simulink model "ASG_collision_avoidance"  (R2024a)
settings: Solver=ode1  StartTime=0.0  StopTime=30  FixedStep=0.01  RelTol=1e-3
libraries: simulink x3
(part 1 of 3)
settings Model: Creator=victo  LastModifiedBy=victo

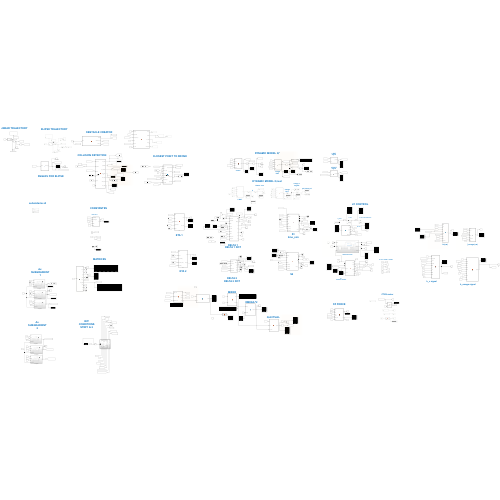
[thumbnail: Simulink's stored preview of the top-level diagram]
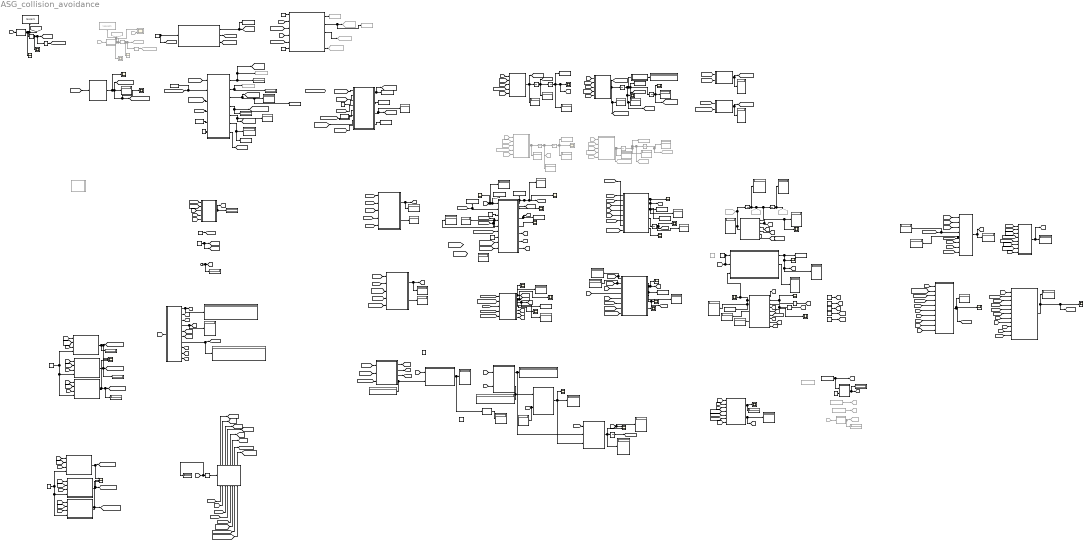
== system ASG_collision_avoidance ==
  note: LOW PASS FILTER
  note: DYNAMIC MODEL Q real
  note: h_omega signal
  note: ANGLES FOR ELIPSE
  note: CONSTANTES
  note: Av. SUBGRADIENT 2
  note: DELTA 1
      | DELTA 1 DOT
  note: ETA 2
  note: ELIPSE TRAJECTORY
  note: S2
  note: U1
      | CONTROL SIGNAL
  note: S1
  note: ETA 1
  note: h_v signal
  note: U1 CONTROL
  note: RHO & K1
  note: S1
      | time_sim
  note: q_dot
  note: f_omega(v,w)
  note: S1
  note: INIT CONDITIONS
      | STEP1 & 2
  note: MATRICES
  note: omega DOT
  note: V DOT
  note: V DOT
  note: Av. SUBGRADIENT 1
  note: omega DOT
  note: Q = Q*
  note: K1, K2, THETA1, THETA2
  note: DYNAMIC MODEL Q*
  note: Kappa - pos
  note: omega, v angular
  note: phi, theta, psi
  note: q = [x,y,z,phi,theta,psi]
  note: q_ddot
  note: subsistema s3
  note: MIXER
  note: OMEGA^2
  note: CTES motor
  note: fv(v,w)
  note: q DOT signal
  note: Q ACTUAL
  note: FZ FORCE
  note: q DDOT signal
  note: V
  note: OBSTACLE CREATOR
  note: COLLISION DETECTION
  note: DELTA 2
      | DELTA 2 DOT
  note: LINEAR TRAJECTORY
  note: CLOSEST POINT TO DRONE
  AverageBlock : Subsystem
  AverageBlock1 : Subsystem
  AverageBlock2 : Subsystem
  AverageBlock3 : Subsystem
  AverageBlock4 : Subsystem
  AverageBlock5 : Subsystem
  Clock : Clock
  Compare To Constant : simulink/Logic and Bit Operations/Compare To Constant  relop===  const=0.0  OutDataTypeStr=boolean
  Constant : Constant  Value=0.5
  Constant1 : Constant  Value=[0;0;0]
  Constant{9..10,19..20} (4 alike) : Constant
  Constant11 : Constant  Value=7
  Constant12 : Constant  Value=pi/4
  Constant13 : Constant  Value=1e-6
  Constant14 : Constant  Commented=on  Value=2*10^(-4)
  Constant15 : Constant  Commented=on  Value=1.95*10^(-4)  VectorParams1D=off
  Constant16 : Constant  Value=5  VectorParams1D=off
  Constant17 : Constant  Commented=on  Value=6*10^(-4)
  Constant18 : Constant  Value=5
  Constant2 : Constant  Value=[1;1;1;1]
  Constant21 : Constant  Value=90
  Constant22 : Constant  Value=7
  Constant3 : Constant  Value=[0;0;6;0;0;0]
  Constant4 : Constant  Value=5  VectorParams1D=off
  Constant5 : Constant  Value=0.03
  Constant6 : Constant  Value=45
  Constant7 : Constant  Value=6*10^(-3)
  Constant8 : Constant  Value=5
  DELTA 1 : Scope
  DELTA 2 : Scope
  DELTA1_DOT : Scope
  DELTA2 DOT4 : Scope
  Derivative1 : Derivative  Commented=on
  Derivative2 : Derivative  Commented=on
  Derivative3 : Derivative
  Derivative4 : Derivative
  Display{,1..54,56..62,64..65,67..69,71,89} (69 alike) : Display
  Display{55,70,73..75,77..78} (7 alike) : Display  Commented=on
  Enabled Subsystem : Subsystem  TreatAsAtomicUnit=on
  From100 : From  Commented=on  GotoTag=KAPPA
  From125 : From  Commented=on  GotoTag=FV
  From126 : From  Commented=on  GotoTag=ZERO_I
  From133 : From  Commented=on  GotoTag=TIME
  From134 : From  Commented=on  GotoTag=I_ZERO
  From146 : From  Commented=on  GotoTag=D_INV
  From147 : From  Commented=on  GotoTag=Q_ACTUAL
  From148 : From  Commented=on  GotoTag=XIsubk
  From157 : From  Commented=on  GotoTag=FW
  From199 : From  Commented=on  GotoTag=JM
  From217 : From  Commented=on  GotoTag=D_INV
  From218 : From  Commented=on  GotoTag=Q_ACTUAL
  From219 : From  Commented=on  GotoTag=XIsubk
  Fz : Scope
  Goto103 : Goto  Commented=on  GotoTag=DM
  Goto104 : Goto  Commented=on  GotoTag=JM
  Goto105 : Goto  Commented=on  GotoTag=JM_INV
  Goto138 : Goto  Commented=on  GotoTag=ANGLES_Q_DOT
  Goto139 : Goto  Commented=on  GotoTag=ANGLES_Q_DDOT
  Goto140 : Goto  Commented=on  GotoTag=V_LIN
  Goto37 : Goto  Commented=on  GotoTag=q_signal
  Goto38 : Goto  Commented=on  GotoTag=q_dot_signal
  Goto47 : Goto  Commented=on  GotoTag=ANGLES_Q
  Goto63 : Goto  Commented=on  GotoTag=q_ddot_signal
  Goto72 : Goto  Commented=on  GotoTag=V_DESEADA
  Goto73 : Goto  Commented=on  GotoTag=KAPPA_TRY
  Goto74 : Goto  Commented=on  GotoTag=V_DOT_DESEADA
  Goto84 : Goto  Commented=on  GotoTag=XI_VALUE
  Goto85 : Goto  Commented=on  GotoTag=OBS_unit_vector
  Goto89 : Goto  Commented=on  GotoTag=CENTER_closest
  HV : Scope
  HW : Scope
  Integrator{,1..6} (7 alike) : Integrator
  Integrator{9..12} (4 alike) : Integrator  Commented=on
  KAPPA : Scope
  KAPPA POS DESEADA : Scope  Commented=on
  KAPPA POS DESEADA1 : Scope
  KAPPA REAL1 : Scope
  KAPPA REAL2 : Scope  Commented=on
  KAPPA des : Scope  Commented=on  NumInputPorts=2
  MATLAB Function : MATLAB Function  TreatAsAtomicUnit=on
  MATLAB Function1 : MATLAB Function  TreatAsAtomicUnit=on
  MATLAB Function10 : MATLAB Function  TreatAsAtomicUnit=on
  MATLAB Function11 : MATLAB Function  TreatAsAtomicUnit=on
  MATLAB Function12 : MATLAB Function  TreatAsAtomicUnit=on
  MATLAB Function13 : MATLAB Function  TreatAsAtomicUnit=on
  MATLAB Function14 : MATLAB Function  TreatAsAtomicUnit=on
  MATLAB Function15 : MATLAB Function  TreatAsAtomicUnit=on
  MATLAB Function16 : MATLAB Function  TreatAsAtomicUnit=on
  MATLAB Function17 : MATLAB Function  TreatAsAtomicUnit=on
  MATLAB Function18 : MATLAB Function  TreatAsAtomicUnit=on
  MATLAB Function19 : MATLAB Function  TreatAsAtomicUnit=on
  MATLAB Function2 : MATLAB Function  TreatAsAtomicUnit=on
  MATLAB Function20 : MATLAB Function  Commented=on  TreatAsAtomicUnit=on
  MATLAB Function21 : MATLAB Function  TreatAsAtomicUnit=on
  MATLAB Function22 : MATLAB Function  TreatAsAtomicUnit=on
  MATLAB Function23 : MATLAB Function  TreatAsAtomicUnit=on
  MATLAB Function24 : MATLAB Function  TreatAsAtomicUnit=on
  MATLAB Function25 : MATLAB Function  TreatAsAtomicUnit=on
  MATLAB Function26 : MATLAB Function  Commented=on  TreatAsAtomicUnit=on
  MATLAB Function27 : MATLAB Function  TreatAsAtomicUnit=on
  MATLAB Function28 : MATLAB Function  Commented=on  TreatAsAtomicUnit=on
  MATLAB Function29 : MATLAB Function  TreatAsAtomicUnit=on
  MATLAB Function3 : MATLAB Function  TreatAsAtomicUnit=on
  MATLAB Function30 : MATLAB Function  TreatAsAtomicUnit=on
  MATLAB Function31 : MATLAB Function  TreatAsAtomicUnit=on
  MATLAB Function32 : MATLAB Function  TreatAsAtomicUnit=on
  MATLAB Function33 : MATLAB Function  TreatAsAtomicUnit=on
  MATLAB Function4 : MATLAB Function  TreatAsAtomicUnit=on
  MATLAB Function45 : MATLAB Function  TreatAsAtomicUnit=on
  MATLAB Function5 : MATLAB Function  Commented=on  TreatAsAtomicUnit=on
  MATLAB Function6 : MATLAB Function  TreatAsAtomicUnit=on
  MATLAB Function7 : MATLAB Function  TreatAsAtomicUnit=on
  MATLAB Function8 : MATLAB Function  TreatAsAtomicUnit=on
  MATLAB Function9 : MATLAB Function  TreatAsAtomicUnit=on
  MIU1 : Constant  Value=0.02
  MIU2 : Constant  Commented=on  Value=0.1
  NORM D1 : Scope
  NORM S1 : Scope
  NORM S2 : Scope
  Norm D2 : Scope
  Q FILTRADA = Q ESTRELLA : Scope
  "Q SIGNAL " : Scope
  Q_comparing : Scope  NumInputPorts=2
  ROTORS VEL : Scope
  S1 : Scope
  S2 : Scope
  SIGN : Signum
  SIGN S1 : Scope
  SIGN S2 : Scope
  Scope : Scope
  Scope1 : Scope  NumInputPorts=3
  Scope2 : Scope  NumInputPorts=3
  Scope3 : Scope
  Scope4 : Scope
  Sign1 : Signum
  Subsystem : Subsystem
  Subsystem1 : Subsystem  Commented=on
  THETA DESIRED : Scope
  THETA DOT DESIRED : Scope
  To Workspace : ToWorkspace  VariableName=dronepos  SampleTime=-1
  To Workspace1 : ToWorkspace  VariableName=simout1  SampleTime=-1
  To Workspace10 : ToWorkspace  VariableName=u1  SaveFormat=Timeseries  SampleTime=-1
  To Workspace11 : ToWorkspace  Commented=on  VariableName=kappad1  SampleTime=-1
  To Workspace12 : ToWorkspace  VariableName=obstaculos  SampleTime=-1
  To Workspace13 : ToWorkspace  VariableName=q_star  SampleTime=-1
  To Workspace14 : ToWorkspace  Commented=on  VariableName=droneor1  SampleTime=-1
  To Workspace15 : ToWorkspace  Commented=on  VariableName=dronepos1  SampleTime=-1
  To Workspace16 : ToWorkspace  Commented=on  VariableName=collision  SampleTime=-1
  To Workspace17 : ToWorkspace  Commented=on  VariableName=idx_obstac  SampleTime=-1
  To Workspace18 : ToWorkspace  Commented=on  VariableName=collision  SampleTime=-1
  To Workspace19 : ToWorkspace  VariableName=kappad1  SampleTime=-1
  To Workspace2 : ToWorkspace  VariableName=s1  SampleTime=-1
  To Workspace20 : ToWorkspace  Commented=on  VariableName=idx_obstac  SampleTime=-1
  To Workspace21 : ToWorkspace  VariableName=forward_vector  SampleTime=-1
  To Workspace22 : ToWorkspace  VariableName=closest_point  SampleTime=-1
  To Workspace23 : ToWorkspace  VariableName=closest_point1  SampleTime=-1
  To Workspace24 : ToWorkspace  VariableName=collision  SampleTime=-1
  To Workspace25 : ToWorkspace  VariableName=idx_obstac  SampleTime=-1
  To Workspace3 : ToWorkspace  VariableName=time_sim  SampleTime=-1
  To Workspace4 : ToWorkspace  VariableName=kappad  SampleTime=-1
  To Workspace5 : ToWorkspace  VariableName=a1  SampleTime=-1
  To Workspace6 : ToWorkspace  VariableName=realkappa  SampleTime=-1
  To Workspace7 : ToWorkspace  VariableName=droneor  SampleTime=-1
  To Workspace8 : ToWorkspace  VariableName=a2  SampleTime=-1
  To Workspace9 : ToWorkspace  VariableName=s2  SampleTime=-1
  Unit Delay : UnitDelay  SampleTime=-1  HasFrameUpgradeWarning=on
  VEL DESEADA : Scope  Commented=on
  VEL DESEADA1 : Scope
  ZETA1 : Scope
  ZETA2 : Scope
  eta1 : MATLAB Function  TreatAsAtomicUnit=on
  eta2 : MATLAB Function  TreatAsAtomicUnit=on
  theta1 : Constant  Value=0.01
  theta2 : Constant  Value=0.5
  theta5 : Constant  Value=1e-6
  wires:
  [C_q] -> MATLAB Function/4(C_q)
  Integrator10/1 -> To Workspace14/1, Goto138/1, Integrator12/1, Display74/1
  [DESIRED_DTHETA_ELIP] -> MATLAB Function8/5(omega_desired)
  MATLAB Function15/1(R) -> [R3]
  MATLAB Function22/1(Q4x1) -> Display47/1
  [q_dot_signal] -> MATLAB Function24/4(q_dot)
  [A2X_AVERAGE] -> MATLAB Function19/6(a2x_average)
  Derivative2/1 -> Goto74/1
  From126/1 -> MATLAB Function28/2(zero_I)
  Enabled Subsystem/5(theta0) -> [THETA0]
  MATLAB Function24/2(Q4) -> [Q4], Display46/1
  [D_INV] -> MATLAB Function14/3(D_inv)
  [THETADOT_DES0] -> eta2/5(THETA_DOT_0)
  MATLAB Function18/1(h_omega) -> [H_OMEGA], HW/1, Display35/1
  [TIME] -> Compare To Constant/1, Display51/1
  MATLAB Function9/7(drag_matrix) -> Display53/1, [DRAG_MATRIX]
  MATLAB Function3/3(a1) -> [A1], To Workspace5/1
  [A1_Z] -> AverageBlock2/1(a1_z)
  MATLAB Function6/1(s1) -> Display10/1, To Workspace2/1, [S1], S1/1
  [D_INV] -> MATLAB Function10/2(D_inv)
  [Q4] -> Display49/1, MATLAB Function2/2(control4x1)
  [THETADOT0] -> eta2/4(THETA_DOT_desired_0)
  MATLAB Function9/9(M) -> [Masa]
  Subsystem/1(Q_STAR) -> [Q], Display64/1, Q FILTRADA = Q ESTRELLA/1, To Workspace13/1
  MATLAB Function3/1(delta1) -> DELTA 1/1, Display11/1, [DELTA1], To Workspace1/1
  [Q] -> MATLAB Function13/1(Q)
  Unit Delay/1 -> [Q_actual]
  From125/1 -> MATLAB Function5/1(fv)
  [V_ACTUAL] -> MATLAB Function45/1(v_lin)
  MATLAB Function13/1(Q_6X1) -> MATLAB Function22/1(Q6x1), Display32/1
  [KA] -> MATLAB Function9/1("Ka ")
  [D_INV] -> MATLAB Function/3(D_inv)
  From199/1 -> MATLAB Function26/1(Jm)
  [OMEGA_ACTV1] -> MATLAB Function45/2(v_ang)
  [DESIRED_DTHETA_ELIP] -> Enabled Subsystem/8(thetadot_desired)
  [THETA1] -> MATLAB Function16/5(theta1)
  Integrator4/1 -> MATLAB Function7/1(vector_rpy), Integrator6/1, To Workspace7/1, [OMEGA_ACTV1], Scope3/1, [ANGLES_Q_DOT], Display21/1
  MATLAB Function15/3(R_ddot) -> [R3_DDOT]
  [V_DESIRED0] -> eta1/3(v_deseada_0)
  MATLAB Function23/1(Q_actual) -> Unit Delay/1, Q_comparing/2, Display37/1
  [D_INV] -> MATLAB Function17/3(D_inv)
  [V_DOT_DESEADA] -> MATLAB Function16/2(v_dot_deseada)
  Enabled Subsystem/2(kappa0) -> [KAPPA_0]
  [V_ACTUAL] -> Enabled Subsystem/1(v_actual)
  Clock/1 -> Display52/1, [TIME]
  Enabled Subsystem/4(kappaD0) -> [KAPPAD0]
  MATLAB Function4/1(k1) -> Display12/1, [K1]
  [THETA2] -> MATLAB Function19/5(theta2)
  [ETA2] -> MATLAB Function18/4(eta2)
  [THETA2] -> AverageBlock5/2(theta)
  [FV] -> MATLAB Function14/1(fv)
  From133/1 -> MATLAB Function20/1(t)
  MATLAB Function28/1(omega_dot) -> Integrator10/1, Display75/1, Goto139/1
  [V_DESEADA] -> Enabled Subsystem/3(v_desired)
  [OMEGA_ACTV1] -> MATLAB Function11/5(omega)
  MATLAB Function12/3(value_s2) -> Display71/1
  MATLAB Function19/3(norm_s2) -> NORM S2/1
  [DRAG_MATRIX] -> MATLAB Function10/8(drag_matrix)
  MATLAB Function8/6(a2_y) -> [A2_Y]
  [V_ACTUAL] -> Display14/1, MATLAB Function3/4(v_actual)
  From148/1 -> MATLAB Function5/5(xi_subv)
  MATLAB Function19/2(Z2) -> [ZETA2], ZETA2/1
  MATLAB Function12/2(value_s1) -> Display68/1
  Constant10/1 -> AverageBlock3/4(constant sign), AverageBlock5/4(constant sign), AverageBlock4/4(constant sign)
  MATLAB Function8/5(a2_x) -> [A2_X]
  Integrator9/1 -> Goto140/1, Integrator11/1, Display70/1
  From157/1 -> MATLAB Function28/1(fw)
  [H_V] -> MATLAB Function12/5(h_v)
  MATLAB Function8/7(a2_z) -> [A2_Z]
  [Q] -> MATLAB Function18/10(Q)
  [TIME] -> AverageBlock1/3(t)
  MATLAB Function9/10(g) -> [G_cte]
  [DRAG_MATRIX] -> MATLAB Function/6(drag_matrix)
  Enabled Subsystem/7(theta_desired0) -> [THETA_DES0]
  [DELTA1] -> MATLAB Function6/1(delta1)
  MATLAB Function8/4(F_d2) -> Norm D2/1
  [ZERO_I] -> MATLAB Function17/2(zero_I)
  MATLAB Function8/2(delta2_dot) -> Display39/1, DELTA2 DOT4/1, [DELTA2_DOT]
  [G_Q] -> MATLAB Function11/6(g_q)
  Derivative1/1 -> VEL DESEADA/1, Goto72/1, Derivative2/1
  [KA] -> MATLAB Function24/3(Ka)
  From219/1 -> MATLAB Function28/5(xi_subw)
  [D] -> MATLAB Function12/1(D)
  [G_Q] -> MATLAB Function/5(g_q)
  [G_cte] -> MATLAB Function24/2(g)
  From147/1 -> MATLAB Function5/4(Q)
  MATLAB Function12/1(u1) -> To Workspace10/1, Display43/1, "Q SIGNAL "/1, Subsystem/3(U1)
  SIGN/1 -> MATLAB Function12/2(sign_s1), SIGN S1/1
  [A2_X] -> AverageBlock3/1(a2_x)
  [A2Z_AVERAGE] -> MATLAB Function19/8(a2z_average)
  [XIsubk] -> MATLAB Function4/1(xi_subkappa)
  [D_INV] -> MATLAB Function18/9(D_inv)
  [TIME] -> AverageBlock3/3(t)
  [Masa] -> MATLAB Function24/1(M)
  [TIME] -> MATLAB Function4/3(t)
  Integrator1/1 -> Display3/1, Goto37/1
  MATLAB Function20/1(kappa) -> KAPPA des/1, Derivative1/1, To Workspace11/1, Goto73/1, KAPPA POS DESEADA/1
  [A2_Y] -> AverageBlock4/1(In1)
  MATLAB Function9/8(l_arm) -> [L_ARM]
  [Q] -> Q_comparing/1, Display48/1
  [Q] -> MATLAB Function/2(Q), Scope/1, Display67/1
  [OMEGA_ACTV1] -> Display18/1, MATLAB Function10/5(omega)
  [V_ACT_0] -> eta1/2(v_0)
  [ZERO_I] -> MATLAB Function18/11(zero_I)
  [DELTA2] -> MATLAB Function18/3(delta2)
  [THETA1] -> AverageBlock1/2(theta)
  From100/1 -> KAPPA des/2
  [RHO1] -> MATLAB Function4/5(rho1)
  [V_ACTUAL] -> MATLAB Function11/4(v)
  [DELTA2] -> MATLAB Function19/1(delta2), Display7/1
  [V_DOT_ACTUAL] -> MATLAB Function25/1(v_lin)
  [V_ACTUAL] -> MATLAB Function16/3(v_actual)
  MATLAB Function25/1(q_dot_signal) -> Display44/1, [q_ddot_signal]
  [KAPPA_TRY] -> To Workspace4/1, MATLAB Function3/2(kappa_desired)
  [I_ZERO] -> MATLAB Function10/1(I_zero)
  AverageBlock5/1(Out1) -> [A2Z_AVERAGE], Scope2/3
  [ZETA2] -> MATLAB Function18/5(zeta2)
  MATLAB Function7/1(R_graph) -> Display26/1
  [THETA1] -> AverageBlock/2(theta)
  [TIME] -> MATLAB Function19/4(t)
  [A2] -> MATLAB Function18/8(a2)
  theta1/1 -> [THETA1]
  [EPSILON] -> MATLAB Function8/3(epsilon)
  eta1/1(eta1) -> [ETA1], Display5/1
  AverageBlock1/1(Out1) -> Scope1/2, Display29/1, [A1Y_AVERAGE]
  From146/1 -> MATLAB Function5/3(D_inv)
  MATLAB Function9/2(D_inv) -> [D_INV]
  [ANGLES_Q_DDOT] -> MATLAB Function25/2(v_ang)
  From134/1 -> MATLAB Function5/2(I_zero)
  [XIsubk] -> MATLAB Function17/5(xi_subw)
  Constant9/1 -> AverageBlock2/4(constant sign), AverageBlock1/4(constant sign), AverageBlock/4(constant sign)
  [G_Q] -> MATLAB Function10/6(g_q)
  [THETA1] -> MATLAB Function4/4(theta1)
  [KAPPA] -> Enabled Subsystem/2(kappa)
  [A1_X] -> AverageBlock/1(a1_x)
  [THETA_DES0] -> eta2/3(THETA_deseada_0)
  [DELTA2_DOT] -> Display65/1, MATLAB Function19/2(delta2_dot)
  AverageBlock4/1(Out1) -> [A2Y_AVERAGE], Scope2/2
  MATLAB Function9/5(I_zero) -> [I_ZERO]
  MATLAB Function1/2(mixer_inv) -> MATLAB Function2/1(mixer_inv), Display15/1
  [FW] -> MATLAB Function18/1(fw)
  [THETA1] -> AverageBlock2/2(theta)
  [DESIRED_THETA_ELIP] -> Enabled Subsystem/7(theta_desired)
  MATLAB Function10/1(fv) -> [FV], Display23/1
  eta2/2(sum_result) -> Display41/1
  [A2_Z] -> AverageBlock5/1(In1)
  [H_OMEGA] -> MATLAB Function12/6(h_omega)
  [KAPPA_0] -> eta1/5(kappa_0)
  MATLAB Function2/1(rotors_vel) -> MATLAB Function23/3(rotors_vel4x1), ROTORS VEL/1, Display34/1
  Constant1/1 -> [XIsubk], [XIsubk_dot]
  MATLAB Function9/4(g_q) -> Display27/1, [G_Q]
  MATLAB Function9/3(C) -> [C_q]
  [TIME] -> AverageBlock4/3(t)
  [Q] -> MATLAB Function17/4(Q)
  [DELTA1_DOT] -> MATLAB Function6/2(delta1_dot)
  [THETA0] -> eta2/2(THETA_0)
  From218/1 -> MATLAB Function28/4(Q)
  [Q] -> MATLAB Function14/4(Q)
  [FV] -> MATLAB Function16/1(fv)
  MATLAB Function6/4(norm_s1) -> NORM S1/1
  Integrator2/1 -> Display/1, ZETA1/1, [ZETA1]
  [XIsubk] -> MATLAB Function14/5(xi_subv)
  [FW] -> MATLAB Function17/1(fw)
  Integrator12/1 -> Goto47/1, Display77/1
  Subsystem/2(Q_DOT_STAR) -> Display69/1
  [q_ddot_signal] -> MATLAB Function24/5(q_ddot)
  [TIME] -> MATLAB Function18/7(t)
  [THETA_ACTUAL] -> MATLAB Function8/1(theta_actual)
  [THETA2] -> AverageBlock4/2(theta)
  AverageBlock2/1(Out1) -> Display1/1, [A1Z_AVERAGE], Scope1/3
  MATLAB Function21/1(desired_theta) -> THETA DESIRED/1, [DESIRED_THETA_ELIP], THETA DOT DESIRED/1, [DESIRED_DTHETA_ELIP], Display13/1
  MATLAB Function8/1(delta2) -> DELTA 2/1, Display38/1, [DELTA2]
  [S1] -> MATLAB Function12/8(s1)
  [TIME] -> AverageBlock2/3(t)
  [TIME] -> MATLAB Function16/10(t)
  MATLAB Function24/1(Fz) -> Display45/1, Fz/1
  [A1_Y] -> AverageBlock1/1(In1)
  MATLAB Function8/3(a2) -> To Workspace8/1, [A2]
  From217/1 -> MATLAB Function28/3(D_inv)
  MATLAB Function16/1(hv) -> [H_V], Display36/1, HV/1
  AverageBlock/1(Out1) -> Display33/1, [A1X_AVERAGE], Scope1/1
  [S1] -> SIGN/1
  Enabled Subsystem/8(thetadot_desired0) -> [THETADOT_DES0]
  [ETA1] -> MATLAB Function6/3(eta1)
  Enabled Subsystem/3(vdesired0) -> [V_DESIRED0]
  Enabled Subsystem/6(thetadot0) -> [THETADOT0]
  [KFC0] -> MATLAB Function11/8(Kf_c0)
  [DESIRED_THETA_ELIP] -> MATLAB Function8/2(theta_desired)
  [C_q] -> MATLAB Function11/3(C)
  [I_ZERO] -> MATLAB Function14/2(I_zero)
  [ANGLES_Q_DDOT] -> MATLAB Function15/3(anglesddot_vector)
  [XIsubk_dot] -> MATLAB Function4/2(xi_subkappa_dot)
  [OMEGA_ACTV1] -> MATLAB Function8/4(omega_actual)
  MATLAB Function5/1(v_dot) -> Integrator9/1, Display73/1
  [RHO2] -> MATLAB Function12/7(k2)
  MATLAB Function3/5(a1_x) -> [A1_X]
  [V_DESEADA] -> MATLAB Function3/5(v_desired), Display30/1
  [S2] -> Sign1/1
  [THETA2] -> eta2/1(theta2)
  [DELTA1] -> MATLAB Function16/8(delta1)
  eta2/1(eta2) -> [ETA2], Display40/1
  [A1X_AVERAGE] -> MATLAB Function6/6(a1x_average)
  MATLAB Function9/6(zero_I) -> [ZERO_I]
  [KAPPA_TRY] -> Enabled Subsystem/4(kappa_try)
  [ZETA1] -> MATLAB Function16/9(zeta1)
  [THETA1] -> eta1/1(theta1)
  MATLAB Function27/1(Km) -> Display50/1, [KM]
  [THETA_ACTUAL] -> Enabled Subsystem/5(theta_actual)
  MATLAB Function11/1(fw) -> Display19/1, [FW]
  MATLAB Function3/4(F_d1) -> NORM D1/1
  [THETA2] -> MATLAB Function18/6(theta2)
  [THETA2] -> AverageBlock3/2(theta)
  MATLAB Function3/6(a1_y) -> [A1_Y]
  MATLAB Function1/1(mixer) -> MATLAB Function23/2(mixer), Display8/1
  MATLAB Function15/4(R_inv) -> MATLAB Function13/2(R_inv), Display22/1
  MIU1/1 -> [MIU], Subsystem/2(MIU2), Subsystem/1(MIU1)
  Integrator/1 -> Display4/1, Goto38/1, MATLAB Function/1(q_dot), Integrator1/1
  [THETA_ACTUAL] -> MATLAB Function15/1(angles_vector)
  [ETA1] -> MATLAB Function16/7(eta1)
  Sign1/1 -> SIGN S2/1, MATLAB Function12/3(sign_s2)
  [DRAG_MATRIX] -> MATLAB Function11/7(drag_matrix)
  Integrator6/1 -> Scope4/1, [THETA_ACTUAL], Display28/1
  MATLAB Function17/1(omega_dot) -> [THETA_ACTUAL_DDOT], [ANGLES_Q_DDOT], Display25/1, Integrator4/1
  MATLAB Function14/1(v_dot) -> [V_DOT_ACTUAL], Display20/1, Integrator3/1
  [ANGLES_Q_DOT] -> MATLAB Function15/2(anglesdot_vector)
  [TIME] -> AverageBlock/3(t)
  MATLAB Function6/3(Z1) -> Integrator2/1
  eta1/2(sum_result) -> Display9/1
  [V_DESEADA] -> MATLAB Function21/1(des_vel)
  [OMEGA_ACTV1] -> Enabled Subsystem/6(omega_actual)
  Enabled Subsystem/1(v_actual0) -> [V_ACT_0]
  [TIME] -> AverageBlock5/3(t)
  [A2Y_AVERAGE] -> MATLAB Function19/7(a2y_average)
  AverageBlock3/1(Out1) -> [A2X_AVERAGE], Scope2/1
  MATLAB Function15/2(R_dot) -> [R3_DOT]
  theta2/1 -> [THETA2]
  [KV] -> MATLAB Function1/1(Kv)
  MATLAB Function45/1(q_dot_signal) -> Display89/1, [q_dot_signal]
  [KFC0] -> MATLAB Function10/7(kf_c0)
  Integrator11/1 -> To Workspace15/1, KAPPA REAL2/1, Display78/1
  [ZERO_I] -> MATLAB Function11/1(zero_I)
  [TIME] -> MATLAB Function6/4(t)
  [D_INV] -> MATLAB Function11/2(D_inv)
  [KM] -> MATLAB Function1/2(Km)
  Compare To Constant/1 -> Enabled Subsystem/Enable
  [A1Y_AVERAGE] -> MATLAB Function6/7(a1y_average)
  [KAPPA] -> KAPPA/1, Display6/1, To Workspace6/1, MATLAB Function3/1(kappa_actual)
  Integrator5/1 -> [KAPPA], KAPPA REAL1/1, Display31/1, To Workspace/1
  [OMEGA_ACTV1] -> MATLAB Function18/2(omega)
  MATLAB Function6/2(t_s1) -> To Workspace3/1
  [V_DESEADA] -> MATLAB Function16/4(v_deseada)
  Constant15/1 -> Goto104/1
  Constant7/1 -> MATLAB Function27/1(Kv), [KV]
  [A1Z_AVERAGE] -> MATLAB Function6/8(a1z_average)
  [C_q] -> MATLAB Function10/3(C)
  Integrator3/1 -> Integrator5/1, Display16/1, [V_ACTUAL]
  [Q] -> MATLAB Function24/7(Q6)
  MATLAB Function3/7(a1_z) -> [A1_Z]
  [K1] -> MATLAB Function12/4(k1)
  [V_ACTUAL] -> Display17/1, MATLAB Function10/4(v)
  MATLAB Function3/2(delta1_dot) -> [DELTA1_DOT], DELTA1_DOT/1
  MATLAB Function/1(out) -> Display2/1, Integrator/1, Goto63/1
  Constant14/1 -> Goto103/1
  MATLAB Function9/1(D) -> Display24/1, [D]
  [A1] -> MATLAB Function16/6(a1)
  MATLAB Function19/1(s2) -> Display42/1, To Workspace9/1, S2/1, [S2]
  theta5/1 -> [EPSILON]
  Constant4/1 -> [RHO2]
  MATLAB Function26/1(Jm_inv) -> Goto105/1, Display55/1
  [THETA1] -> MATLAB Function6/5(theta1)
  [S2] -> MATLAB Function12/9(s2)
  Constant5/1 -> MATLAB Function27/2(porcent_force)
  [ETA2] -> MATLAB Function19/3(eta2)
  [R3] -> MATLAB Function23/1(R)
  Constant/1 -> [KA]
  [KAPPAD0] -> eta1/4(kappa_desired_0)
  [THETA_ACTUAL] -> MATLAB Function24/6(theta_actual)
  MATLAB Function29/1(obstaculos) -> To Workspace12/1, [OBSTACLES]
  [KAPPA] -> MATLAB Function30/1(drone_center)
  [OBSTACLES] -> MATLAB Function30/3(obstacles)
  MATLAB Function30/1(hay_colision) -> [XI_VALUE], To Workspace16/1, Display54/1
  MATLAB Function30/2(idx_obstaculo) -> To Workspace17/1, Display56/1
  [XI_VALUE] -> MATLAB Function3/6(collision)
  Constant8/1 -> MATLAB Function3/7(gamma)
  MATLAB Function30/3(centro_obstaculo) -> To Workspace22/1, Display57/1, [CENTER_closest]
  Constant11/1 -> [MIN_DISTANCE], MATLAB Function30/2(max_distancia)
  MATLAB Function30/4(angulo_relativo) -> Display58/1, [OBST_angle]
  [TIME] -> MATLAB Function31/1(t)
  Derivative4/1 -> [V_DOT_DESEADA]
  Derivative3/1 -> VEL DESEADA1/1, [V_DESEADA], Derivative4/1
  MATLAB Function31/1(kappa) -> KAPPA POS DESEADA1/1, Derivative3/1, To Workspace19/1, [KAPPA_TRY]
  Constant12/1 -> MATLAB Function30/5(fov_angle)
  [THETA_ACTUAL] -> MATLAB Function30/4(drone_angles)
  MATLAB Function30/5(vector_centro) -> [OBS_unit_vector], Display59/1
  Constant13/1 -> MATLAB Function3/3(epsilon)
  Constant19/1 -> MATLAB Function30/6(Kd)
  Constant16/1 -> [RHO1]
  [V_ACTUAL] -> MATLAB Function32/2(kappa_derivative)
  Constant6/1 -> MATLAB Function32/1(FOV_angle)
  [KAPPA] -> MATLAB Function32/4(kappa)
  MATLAB Function29/3(radios_value) -> [RADIOS_VALUE]
  MATLAB Function29/2(obstacles_center_list) -> [OBS_CENTER_LIST]
  [OBS_CENTER_LIST] -> MATLAB Function32/3(obstaculos_center_list)
  [RADIOS_VALUE] -> MATLAB Function32/5(radio_value)
  Constant20/1 -> MATLAB Function32/6(drone_radio)
  MATLAB Function32/2(collision) -> To Workspace18/1, Goto84/1
  MATLAB Function32/1(idx_min) -> To Workspace20/1
  MATLAB Function32/3(unit_vector) -> Goto85/1
  MATLAB Function32/5(closest_center) -> Goto89/1
  MATLAB Function30/6(forward_vector) -> To Workspace21/1, Display60/1
  Constant18/1 -> MATLAB Function29/1(shifft1), [SHIFFT1]
  [KAPPA] -> MATLAB Function33/1(dron_pos)
  [SHIFFT1] -> MATLAB Function33/2(shifft1)
  MATLAB Function33/1(punto_mas_cercano) -> [CENTER_clst], To Workspace23/1
  MATLAB Function33/3(unitary_vector) -> Display62/1, [UNITARY_VEC]
  MATLAB Function33/4(hay_colision) -> To Workspace24/1
  MATLAB Function33/2(idx_obstaculo) -> To Workspace25/1
  [THETA_ACTUAL] -> MATLAB Function33/4(drone_angles)
  Constant21/1 -> MATLAB Function33/5(fov_angle)
  Constant22/1 -> MATLAB Function33/3(distancia_minima)
  [UNITARY_VEC] -> MATLAB Function3/9(unitary_vector)
  [CENTER_clst] -> MATLAB Function3/8(center_closest)
  [OBSTACLES] -> MATLAB Function33/6(obstaculos)
  [CENTER_closest] -> MATLAB Function33/7(center_closest_red)
  MATLAB Function30/7(aux_variable) -> [AUX_VAR]
  [AUX_VAR] -> MATLAB Function33/8(aux_variable)

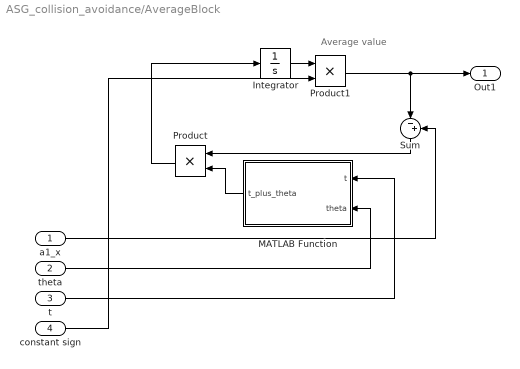
== system ASG_collision_avoidance/AverageBlock ==
  note: Average value
  a1_x : Inport
  theta : Inport  Port=2
  t : Inport  Port=3
  constant sign : Inport  Port=4
  Integrator : Integrator
  MATLAB Function : MATLAB Function  TreatAsAtomicUnit=on
  Product : Product
  Product1 : Product
  Sum : Sum  Inputs=|-+
  Out1 : Outport
  wires:
  MATLAB Function/1(t_plus_theta) -> Product/2
  Sum/1 -> Product/1
  Product/1 -> Integrator/1
  theta/1 -> MATLAB Function/2(theta)
  a1_x/1 -> Sum/2
  t/1 -> MATLAB Function/1(t)
  Integrator/1 -> Product1/1
  Product1/1 -> Out1/1, Sum/1
  constant sign/1 -> Product1/2

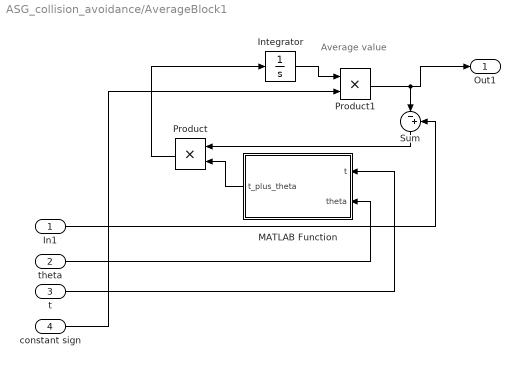
== system ASG_collision_avoidance/AverageBlock1 ==
  note: Average value
  In1 : Inport
  theta : Inport  Port=2
  t : Inport  Port=3
  constant sign : Inport  Port=4
  Integrator : Integrator
  MATLAB Function : MATLAB Function  TreatAsAtomicUnit=on
  Product : Product
  Product1 : Product
  Sum : Sum  Inputs=|-+
  Out1 : Outport
  wires:
  MATLAB Function/1(t_plus_theta) -> Product/2
  Sum/1 -> Product/1
  Product/1 -> Integrator/1
  theta/1 -> MATLAB Function/2(theta)
  In1/1 -> Sum/2
  t/1 -> MATLAB Function/1(t)
  Product1/1 -> Sum/1, Out1/1
  Integrator/1 -> Product1/1
  constant sign/1 -> Product1/2

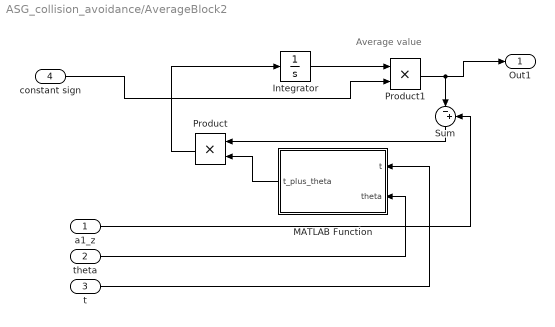
== system ASG_collision_avoidance/AverageBlock2 ==
  note: Average value
  a1_z : Inport
  theta : Inport  Port=2
  t : Inport  Port=3
  constant sign : Inport  Port=4
  Integrator : Integrator
  MATLAB Function : MATLAB Function  TreatAsAtomicUnit=on
  Product : Product
  Product1 : Product
  Sum : Sum  Inputs=|-+
  Out1 : Outport
  wires:
  MATLAB Function/1(t_plus_theta) -> Product/2
  Sum/1 -> Product/1
  Product/1 -> Integrator/1
  theta/1 -> MATLAB Function/2(theta)
  a1_z/1 -> Sum/2
  t/1 -> MATLAB Function/1(t)
  Integrator/1 -> Product1/1
  Product1/1 -> Sum/1, Out1/1
  constant sign/1 -> Product1/2

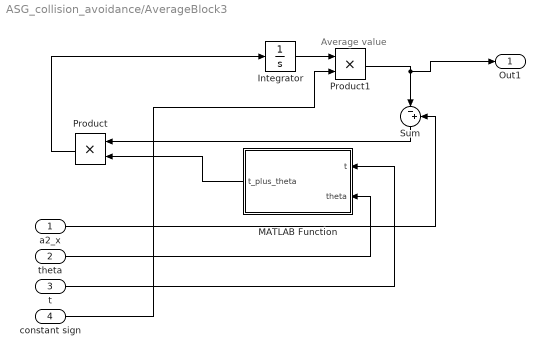
== system ASG_collision_avoidance/AverageBlock3 ==
  note: Average value
  a2_x : Inport
  theta : Inport  Port=2
  t : Inport  Port=3
  constant sign : Inport  Port=4
  Integrator : Integrator
  MATLAB Function : MATLAB Function  TreatAsAtomicUnit=on
  Product : Product
  Product1 : Product
  Sum : Sum  Inputs=|-+
  Out1 : Outport
  wires:
  MATLAB Function/1(t_plus_theta) -> Product/2
  Sum/1 -> Product/1
  Product/1 -> Integrator/1
  theta/1 -> MATLAB Function/2(theta)
  a2_x/1 -> Sum/2
  t/1 -> MATLAB Function/1(t)
  Integrator/1 -> Product1/1
  constant sign/1 -> Product1/2
  Product1/1 -> Sum/1, Out1/1

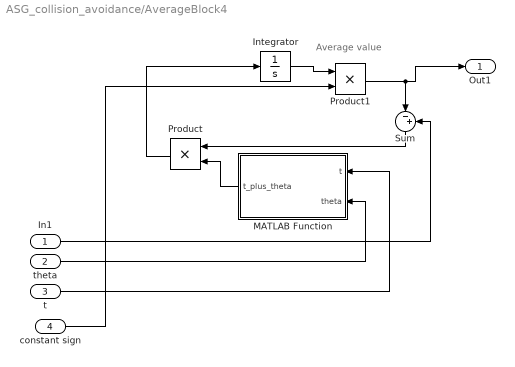
== system ASG_collision_avoidance/AverageBlock4 ==
  note: Average value
  In1 : Inport
  theta : Inport  Port=2
  t : Inport  Port=3
  constant sign : Inport  Port=4
  Integrator : Integrator
  MATLAB Function : MATLAB Function  TreatAsAtomicUnit=on
  Product : Product
  Product1 : Product
  Sum : Sum  Inputs=|-+
  Out1 : Outport
  wires:
  MATLAB Function/1(t_plus_theta) -> Product/2
  Sum/1 -> Product/1
  Product/1 -> Integrator/1
  theta/1 -> MATLAB Function/2(theta)
  In1/1 -> Sum/2
  t/1 -> MATLAB Function/1(t)
  Integrator/1 -> Product1/1
  Product1/1 -> Sum/1, Out1/1
  constant sign/1 -> Product1/2

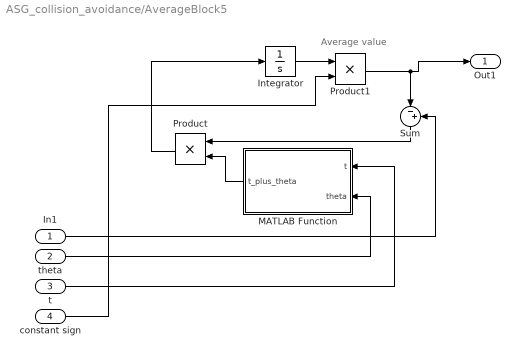
== system ASG_collision_avoidance/AverageBlock5 ==
  note: Average value
  In1 : Inport
  theta : Inport  Port=2
  t : Inport  Port=3
  constant sign : Inport  Port=4
  Integrator : Integrator
  MATLAB Function : MATLAB Function  TreatAsAtomicUnit=on
  Product : Product
  Product1 : Product
  Sum : Sum  Inputs=|-+
  Out1 : Outport
  wires:
  MATLAB Function/1(t_plus_theta) -> Product/2
  Sum/1 -> Product/1
  Product/1 -> Integrator/1
  theta/1 -> MATLAB Function/2(theta)
  In1/1 -> Sum/2
  t/1 -> MATLAB Function/1(t)
  Integrator/1 -> Product1/1
  Product1/1 -> Sum/1, Out1/1
  constant sign/1 -> Product1/2

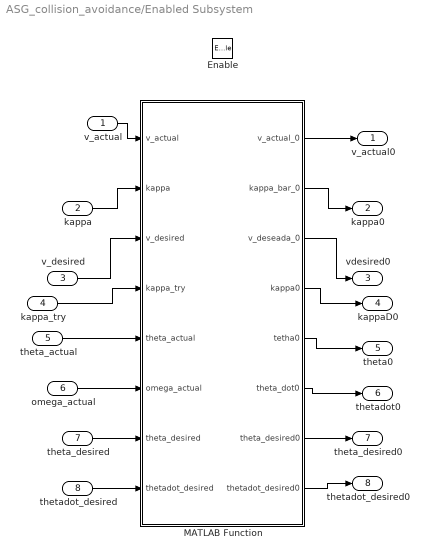
== system ASG_collision_avoidance/Enabled Subsystem ==
  v_actual : Inport
  kappa : Inport  Port=2
  v_desired : Inport  Port=3
  kappa_try : Inport  Port=4
  theta_actual : Inport  Port=5
  omega_actual : Inport  Port=6
  theta_desired : Inport  Port=7
  thetadot_desired : Inport  Port=8
  Enable : EnablePort
  MATLAB Function : MATLAB Function  TreatAsAtomicUnit=on
  v_actual0 : Outport
  kappa0 : Outport  Port=2
  vdesired0 : Outport  Port=3
  kappaD0 : Outport  Port=4
  theta0 : Outport  Port=5
  thetadot0 : Outport  Port=6
  theta_desired0 : Outport  Port=7
  thetadot_desired0 : Outport  Port=8
  wires:
  v_actual/1 -> MATLAB Function/1(v_actual)
  kappa/1 -> MATLAB Function/2(kappa)
  MATLAB Function/2(kappa_bar_0) -> kappa0/1
  MATLAB Function/1(v_actual_0) -> v_actual0/1
  v_desired/1 -> MATLAB Function/3(v_desired)
  MATLAB Function/3(v_deseada_0) -> vdesired0/1
  kappa_try/1 -> MATLAB Function/4(kappa_try)
  MATLAB Function/4(kappa0) -> kappaD0/1
  MATLAB Function/5(tetha0) -> theta0/1
  MATLAB Function/6(theta_dot0) -> thetadot0/1
  theta_actual/1 -> MATLAB Function/5(theta_actual)
  omega_actual/1 -> MATLAB Function/6(omega_actual)
  theta_desired/1 -> MATLAB Function/7(theta_desired)
  thetadot_desired/1 -> MATLAB Function/8(thetadot_desired)
  MATLAB Function/7(theta_desired0) -> theta_desired0/1
  MATLAB Function/8(thetadot_desired0) -> thetadot_desired0/1

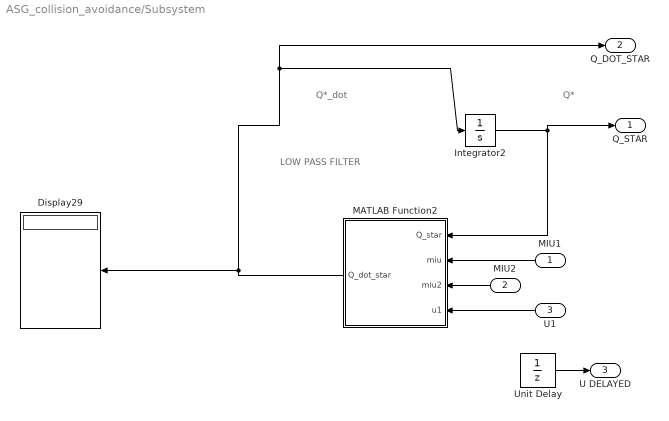
== system ASG_collision_avoidance/Subsystem ==
  note: LOW PASS FILTER
  note: Q*_dot
  note: Q*
  MIU1 : Inport
  MIU2 : Inport  Port=2
  U1 : Inport  Port=3
  Display29 : Display
  Integrator2 : Integrator  UpperSaturationLimit=10  LowerSaturationLimit=-10  IgnoreLimit=on
  MATLAB Function2 : MATLAB Function  TreatAsAtomicUnit=on
  Unit Delay : UnitDelay  SampleTime=-1  HasFrameUpgradeWarning=on
  Q_STAR : Outport
  Q_DOT_STAR : Outport  Port=2
  U DELAYED : Outport  Port=3
  wires:
  MATLAB Function2/1(Q_dot_star) -> Q_DOT_STAR/1, Integrator2/1, Display29/1
  MIU1/1 -> MATLAB Function2/2(miu)
  U1/1 -> MATLAB Function2/4(u1)
  Integrator2/1 -> Q_STAR/1, MATLAB Function2/1(Q_star)
  MIU2/1 -> MATLAB Function2/3(miu2)
  Unit Delay/1 -> U DELAYED/1
